simulink subsystem "Extremum_Seeking_vx_gain"  (R2024a)
settings: Solver=VariableStepAuto  StartTime=0.0  StopTime=10.0  RelTol=1e-3
undefined symbols (not defined in the file): a, C, esc_ic, omega, phi, x_c, x_l
settings Model: Creator=Henrique Mesquita  LastModifiedBy=Henrique Mesquita
settings OptimizationCC: ReuseModelBlockBuffer=off
settings DebuggingCC: UnconnectedInputMsg=warning  UnconnectedOutputMsg=warning  UnconnectedLineMsg=warning
settings ModelReferenceCC: EnableRefExpFcnMdlSchedulingChecks=on
settings RTWCC: GPUComputeCapability=3.5  DLArmComputeVersion=19.05

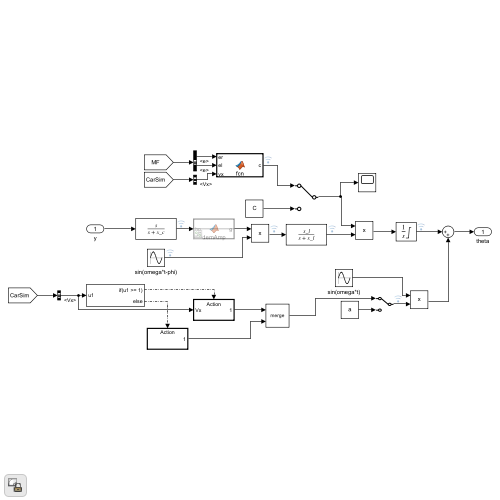
[thumbnail: Simulink's stored preview of the top-level diagram]
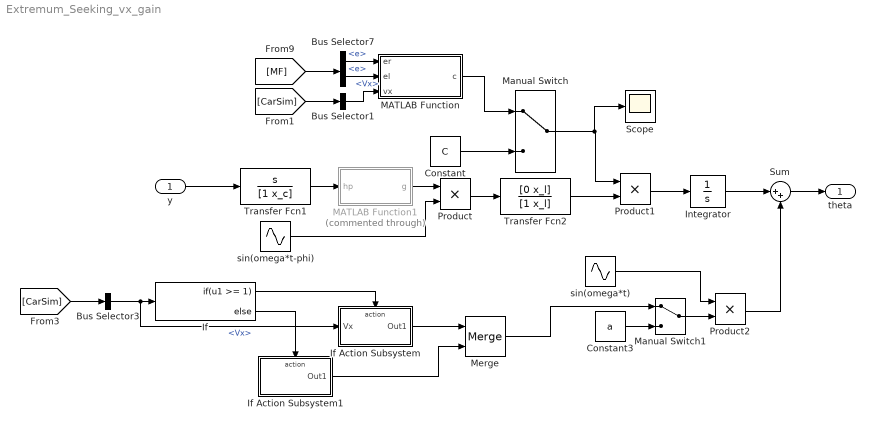
== system Extremum_Seeking_vx_gain ==
  y : Inport
  Bus Selector1 : BusSelector  OutputSignals=Vx
  Bus Selector3 : BusSelector  OutputSignals=Vx
  Bus Selector7 : BusSelector  OutputSignals=info (signal 1).e,info (signal 2).e
  Constant : Constant  Value=C
  Constant3 : Constant  Value=a
  If : If  IfExpression=u1 >= 1
  If Action Subsystem : Subsystem  TreatAsAtomicUnit=on
  If Action Subsystem1 : Subsystem  TreatAsAtomicUnit=on
  Integrator : Integrator  InitialCondition=esc_ic  LimitOutput=on  UpperSaturationLimit=0.2  LowerSaturationLimit=0.015
  MATLAB Function : MATLAB Function  TreatAsAtomicUnit=on
  MATLAB Function1 : MATLAB Function  Commented=through  TreatAsAtomicUnit=on
  Manual Switch : ManualSwitch
  Manual Switch1 : ManualSwitch
  Merge : Merge
  Product : Product
  Product1 : Product
  Product2 : Product
  Scope : Scope
  Sum : Sum  Inputs=|++
  Transfer Fcn1 : TransferFcn  Numerator=[1 0]  Denominator=[1 x_c]
  Transfer Fcn2 : TransferFcn  Numerator=[0 x_l]  Denominator=[1 x_l]
  sin(omega*t) : Sin  Frequency=omega  SampleTime=0
  sin(omega*t-phi) : Sin  Frequency=omega  Phase=phi  SampleTime=0
  theta : Outport
  wires:
  sin(omega*t)/1 -> Product2/1
  Product2/1 -> Sum/2
  Sum/1 -> theta/1
  Product/1 -> Transfer Fcn2/1
  Transfer Fcn2/1 -> Product1/2
  y/1 -> Transfer Fcn1/1
  sin(omega*t-phi)/1 -> Product/2
  Product1/1 -> Integrator/1
  Integrator/1 -> Sum/1
  [MF] -> Bus Selector7/1
  Bus Selector7/1 -> MATLAB Function/1(er)  "<e>"
  Bus Selector7/2 -> MATLAB Function/2(el)  "<e>"
  MATLAB Function/1(c) -> Manual Switch/1
  Constant/1 -> Manual Switch/2
  Manual Switch/1 -> Product1/1, Scope/1
  Transfer Fcn1/1 -> MATLAB Function1/1(hp)
  [CarSim] -> Bus Selector1/1
  Bus Selector1/1 -> MATLAB Function/3(vx)  "<Vx>"
  MATLAB Function1/1(g) -> Product/1
  Manual Switch1/1 -> Product2/2
  Constant3/1 -> Manual Switch1/2
  [CarSim] -> Bus Selector3/1
  Bus Selector3/1 -> If/1, If Action Subsystem/1(Vx)  "<Vx>"
  If Action Subsystem/1(Out1) -> Merge/1
  If Action Subsystem1/1(Out1) -> Merge/2
  If/1 -> If Action Subsystem/Action
  If/2 -> If Action Subsystem1/Action
  Merge/1 -> Manual Switch1/1

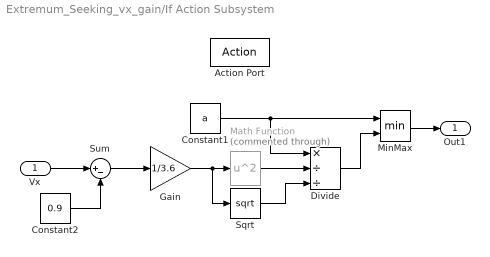
== system Extremum_Seeking_vx_gain/If Action Subsystem ==
  Vx : Inport
  Action Port : ActionPort
  Constant1 : Constant  Value=a
  Constant2 : Constant  Value=0.9
  Divide : Product  Inputs=*//
  Gain : Gain  Gain=1/3.6
  Math Function : Math  Commented=through  Operator=square
  MinMax : MinMax  Inputs=2
  Sqrt : Sqrt
  Sum : Sum  Inputs=|+-
  Out1 : Outport
  wires:
  Sqrt/1 -> Divide/3
  Vx/1 -> Sum/1
  Sum/1 -> Gain/1
  Gain/1 -> Math Function/1, Sqrt/1
  MinMax/1 -> Out1/1
  Divide/1 -> MinMax/2
  Constant2/1 -> Sum/2
  Math Function/1 -> Divide/2
  Constant1/1 -> Divide/1, MinMax/1

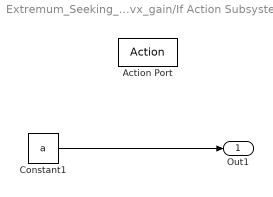
== system Extremum_Seeking_vx_gain/If Action Subsystem1 ==
  Action Port : ActionPort
  Constant1 : Constant  Value=a
  Out1 : Outport
  wires:
  Constant1/1 -> Out1/1

== matlab function Extremum_Seeking_vx_gain/MATLAB Function ==
  data: er input; c output; el input; C parameter; vx input
function c = fcn(er, el, C, vx)

VMAX = 120;
VMIN = 1;

persistent de_ant;
persistent e_ant;
if(isempty(de_ant)||isempty(e_ant))
    de_ant = 0;
    e_ant = 0;
end

e = (er+el)/2;

% if(e^2<1e-4)
%     c = C;
% else
%     c = C*(exp(-(e^2)/0.0001));
% end
% c = C*(exp(-(e^2)/0.01));
% c=C;

if(vx>VMAX || vx<0.1)
    c=0;
else
%     c = min([C (VMAX-vx)/(VMAX-VMIN)*C]);
%     c = min([C exp(-(vx-VMIN)/(VMAX/5))*C]);
%     if c < C/30
%         c = C/30;
%     end
    c = (C/(1+exp((vx-10)/(2)))+0.2);
%     c=C;
%     c = c*(exp(-(e^2)/0.0001));
end
% de = 19.03*(e-e_ant)+0.9048*de_ant;
% 
% if(abs(e)>0.01 || abs(de)>0.05)
%     c=0;
% else
%     c = C;
% end

% if(j<=0)
%     y = 0;
% else
%     y = 200*j;
% end

== matlab function Extremum_Seeking_vx_gain/MATLAB Function1 ==
  data: hp input; g output
function g = demAmp(hp)

% if(abs(hp)>0.05)
%     g = hp*(exp(-(abs(hp)-0.05)/0.01));
% else
%     g = hp;
% end

% g = hp*(exp(-hp^2/0.005));
g = hp;
